simulink model "mi_modelo_MI"  (R2022b)
settings: Solver=VariableStepAuto  StartTime=0.0  StopTime=250  RelTol=1e-3
undefined symbols (not defined in the file): DiscIntNeverNeededParam, fb, fd, J, kt, Lm, Lr, Ls, Rs, sg, Tr
libraries: neural x166
(part 2 of 5)

== system mi_modelo_MI/Motor MI/landa_beta_r ==
  i_beta_s : Inport
  landa_alpha_r : Inport  Port=2
  wr : Inport  Port=3
  1/Tr : Gain  Gain=1/Tr
  Add : Sum  Inputs=++-
  Integrator : Integrator
  Lm/Tr : Gain  Gain=Lm/Tr
  Product : Product
  landa_beta_r : Outport
  wires:
  i_beta_s/1 -> Lm/Tr/1
  Integrator/1 -> landa_beta_r/1, 1/Tr/1
  wr/1 -> Product/2
  landa_alpha_r/1 -> Product/1
  Add/1 -> Integrator/1
  1/Tr/1 -> Add/3
  Lm/Tr/1 -> Add/1
  Product/1 -> Add/2

== system mi_modelo_MI/Motor MI/landa_dr ==
  i_ds : Inport
  landa_qr : Inport  Port=2
  we : Inport  Port=3
  wr : Inport  Port=4
  Gain : Gain  Gain=Lm/Tr
  Gain1 : Gain  Gain=1/Tr
  Integrator : Integrator
  Product : Product
  Subtract : Sum  Inputs=++-
  Subtract1 : Sum  Inputs=+-
  landa_dr : Outport
  wires:
  i_ds/1 -> Gain/1
  Integrator/1 -> Gain1/1, landa_dr/1
  Gain/1 -> Subtract/1
  Gain1/1 -> Subtract/3
  Subtract/1 -> Integrator/1
  landa_qr/1 -> Product/2
  Product/1 -> Subtract/2
  Subtract1/1 -> Product/1
  wr/1 -> Subtract1/2
  we/1 -> Subtract1/1

== system mi_modelo_MI/Motor MI/landa_qr ==
  i_qs : Inport
  landa_dr : Inport  Port=2
  we : Inport  Port=3
  wr : Inport  Port=4
  Gain : Gain  Gain=Lm/Tr
  Gain1 : Gain  Gain=1/Tr
  Integrator : Integrator
  Product : Product
  Subtract : Sum  Inputs=+--
  Subtract1 : Sum  Inputs=+-
  landa_qr : Outport
  wires:
  Gain1/1 -> Subtract/3
  landa_dr/1 -> Product/2
  Product/1 -> Subtract/2
  Subtract1/1 -> Product/1
  Gain/1 -> Subtract/1
  Integrator/1 -> Gain1/1, landa_qr/1
  Subtract/1 -> Integrator/1
  i_qs/1 -> Gain/1
  wr/1 -> Subtract1/2
  we/1 -> Subtract1/1

== system mi_modelo_MI/Motor MI/rotor_speed ==
  Te : Inport
  Tl : Inport  Port=2
  Gain : Gain  Gain=1/J
  Gain1 : Gain  Gain=fd
  Integrator : Integrator
  Subtract : Sum  Inputs=+--
  wr : Outport
  wires:
  Integrator/1 -> Gain1/1, wr/1
  Gain/1 -> Integrator/1
  Te/1 -> Subtract/1
  Subtract/1 -> Gain/1
  Tl/1 -> Subtract/2
  Gain1/1 -> Subtract/3

== system mi_modelo_MI/Motor MI/torque_elec ==
  landa_dr : Inport
  i_qs : Inport  Port=2
  landa_qr : Inport  Port=3
  i_ds : Inport  Port=4
  Gain : Gain  Gain=kt
  Product : Product
  Product1 : Product
  Subtract : Sum  Inputs=+-
  Te : Outport
  wires:
  i_qs/1 -> Product/2
  landa_dr/1 -> Product/1
  landa_qr/1 -> Product1/1
  i_ds/1 -> Product1/2
  Product/1 -> Subtract/1
  Product1/1 -> Subtract/2
  Gain/1 -> Te/1
  Subtract/1 -> Gain/1

== system mi_modelo_MI/NARX WR/Layer 1 ==
  "p{1}" : Inport  PortDimensions=4  SampleTime=1
      mask Display: e = 0.06;c1 = [120 230 180]/255;c2 = ([120 230 180]+0)/(256+128);c3 = ([120 230 180]+128)/(256+128);patch([0 1 1 0],[0 0 1 1],c1);patch([0 1 1 1-e 1-e 0+e],[0 0 1 1-e 0+e 0+e],c2);patch([0 0 1 1-e 0+e 0+e],[0 1 1 1-e 1-e 0+e],c3);plot([0 1 1 0 0],[0 0 1 1 0]);
  "a{2} " : Inport  Port=2  PortDimensions=1  SampleTime=1
      mask Display: e = 0.06;c1 = [120 230 180]/255;c2 = ([120 230 180]+0)/(256+128);c3 = ([120 230 180]+128)/(256+128);patch([0 1 1 0],[0 0 1 1],c1);patch([0 1 1 1-e 1-e 0+e],[0 0 1 1-e 0+e 0+e],c2);patch([0 0 1 1-e 0+e 0+e],[0 1 1 1-e 1-e 0+e],c3);plot([0 1 1 0 0],[0 0 1 1 0]);
  Delays 1 : Subsystem
      mask Display: e = 0.06;c1 = [120 150 230]/255;c2 = ([120 150 230]+0)/383;c3 = ([120 150 230]+128)/383;patch([0 1 1 0],[0 0 1 1],c1);patch([0 1 1 1-e 1-e 0+e],[0 0 1 1-e 0+e 0+e],c2);patch([0 0 1 1-e 0+e 0+e],[0 1 1 1-e 1-e 0+e],c3);plot([0 1 1 0 0],[0 0 1 1 0]);disp('1-2');
  Delays 2 : Subsystem
      mask Display: e = 0.06;c1 = [120 150 230]/255;c2 = ([120 150 230]+0)/383;c3 = ([120 150 230]+128)/383;patch([0 1 1 0],[0 0 1 1],c1);patch([0 1 1 1-e 1-e 0+e],[0 0 1 1-e 0+e 0+e],c2);patch([0 0 1 1-e 0+e 0+e],[0 1 1 1-e 1-e 0+e],c3);plot([0 1 1 0 0],[0 0 1 1 0]);disp('1-2');
  "IW{1,1}" : Subsystem
      mask Display: e = 0.06;c1 = [120 150 230]/255;c2 = ([120 150 230]+0)/383;c3 = ([120 150 230]+128)/383;patch([0 1 1 0],[0 0 1 1],c1);patch([0 1 1 1-e 1-e 0+e],[0 0 1 1-e 0+e 0+e],c2);patch([0 0 1 1-e 0+e 0+e],[0 1 1 1-e 1-e 0+e],c3);plot([0 1 1 0 0],[0 0 1 1 0]);disp('W');
  "LW{1,2}" : Subsystem
      mask Display: e = 0.06;c1 = [120 150 230]/255;c2 = ([120 150 230]+0)/383;c3 = ([120 150 230]+128)/383;patch([0 1 1 0],[0 0 1 1],c1);patch([0 1 1 1-e 1-e 0+e],[0 0 1 1-e 0+e 0+e],c2);patch([0 0 1 1-e 0+e 0+e],[0 1 1 1-e 1-e 0+e],c3);plot([0 1 1 0 0],[0 0 1 1 0]);disp('W');
  "b{1}" : Constant  Value=[-1.8998763615156166739694754141964949667453765869140625;1.7162424238927365127693747126613743603229522705078125;1.873778335719318288710155684384517371654510498046875;1.2761620955153916145974335449864156544208526611328125;-0.943914474908234435446274801506660878658294677734375;0.6149915255390541179991714670904912054538726806640625;1.2780413566537642822140696807764470577239990234375;1.01453395825711556454962192219682037830352783203125;0.842453920367021158455145268817432224750518798828125;0.73720646264958755722318528569303452968597412109375;0.4984224377356063495625448922510258853435516357421875;-0.64613247194810929929786880165920592844486236572265625;-0.1218890242028434489629518111541983671486377716064453125;0.006777158234348323873064146027900278568267822265625;-0.02844198720616673836669718866687617264688014984130859375;0.31303593350495850788917095997021533548831939697265625;-0.57699423755770595789726939983665943145751953125;0.316780417226055988066946156322956085205078125;0.68420763225480529801103557474561966955661773681640625;0.83882619819923254222970854243612848222255706787109375;0.68908943201714423221204697256325744092464447021484375;-0.79636082633369686956115174325532279908657073974609375;0.99883419950671770148886707829660736024379730224609375;-0.96148781215878909023331289063207805156707763671875;-0.888341997791541881923649270902387797832489013671875;1.134062865515947038375088595785200595855712890625;-1.5752696276526256813355075792060233652591705322265625;1.5323125142516909047429862766875885426998138427734375;1.739636071487099311383417443721555173397064208984375;-2.010421496688121312246266825241036713123321533203125]
      mask Display: e = 0.06;c1 = [120 150 230]/255;c2 = ([120 150 230]+0)/383;c3 = ([120 150 230]+128)/383;patch([0 1 1 0],[0 0 1 1],c1);patch([0 1 1 1-e 1-e 0+e],[0 0 1 1-e 0+e 0+e],c2);patch([0 0 1 1-e 0+e 0+e],[0 1 1 1-e 1-e 0+e],c3);plot([0 1 1 0 0],[0 0 1 1 0]);disp('b');
  netsum : Sum  Inputs=3  InputSameDT=on  SaturateOnIntegerOverflow=on  OutDataTypeStr=Inherit: Same as first input
      mask Display: e = 0.06;c1 = [120 150 230]/255;c2 = ([120 150 230]+0)/383;c3 = ([120 150 230]+128)/383;patch([0 1 1 0],[0 0 1 1],c1);patch([0 1 1 1-e 1-e 0+e],[0 0 1 1-e 0+e 0+e],c2);patch([0 0 1 1-e 0+e 0+e],[0 1 1 1-e 1-e 0+e],c3);plot([0 1 1 0 0],[0 0 1 1 0]);disp('+');
  tansig : neural/Transfer Functions/tansig
  "a{1}" : Outport  InitialOutput=[0;0;0;0;0;0;0;0;0;0;0;0;0;0;0;0;0;0;0;0;0;0;0;0;0;0;0;0;0;0]
      mask Display: e = 0.06;c1 = [120 230 180]/255;c2 = ([120 230 180]+0)/(256+128);c3 = ([120 230 180]+128)/(256+128);patch([0 1 1 0],[0 0 1 1],c1);patch([0 1 1 1-e 1-e 0+e],[0 0 1 1-e 0+e 0+e],c2);patch([0 0 1 1-e 0+e 0+e],[0 1 1 1-e 1-e 0+e],c3);plot([0 1 1 0 0],[0 0 1 1 0]);
  wires:
  "p{1}"/1 -> Delays 1/1("p{1}")
  Delays 1/1("pd{1,1}") -> "IW{1,1}"/1("pd{1,1}")
  "IW{1,1}"/1("iz{1,1}") -> netsum/1
  "a{2} "/1 -> Delays 2/1("p{1}")
  Delays 2/1("pd{1,2}") -> "LW{1,2}"/1("ad{1,2}")
  "LW{1,2}"/1("lz{1,2}") -> netsum/2
  "b{1}"/1 -> netsum/3
  netsum/1 -> tansig/1
  tansig/1 -> "a{1}"/1

== system mi_modelo_MI/NARX WR/Layer 2 ==
  "a{1} " : Inport  PortDimensions=30  SampleTime=1
      mask Display: e = 0.06;c1 = [120 230 180]/255;c2 = ([120 230 180]+0)/(256+128);c3 = ([120 230 180]+128)/(256+128);patch([0 1 1 0],[0 0 1 1],c1);patch([0 1 1 1-e 1-e 0+e],[0 0 1 1-e 0+e 0+e],c2);patch([0 0 1 1-e 0+e 0+e],[0 1 1 1-e 1-e 0+e],c3);plot([0 1 1 0 0],[0 0 1 1 0]);
  Delays 1 : Subsystem
      mask Display: e = 0.06;c1 = [120 150 230]/255;c2 = ([120 150 230]+0)/383;c3 = ([120 150 230]+128)/383;patch([0 1 1 0],[0 0 1 1],c1);patch([0 1 1 1-e 1-e 0+e],[0 0 1 1-e 0+e 0+e],c2);patch([0 0 1 1-e 0+e 0+e],[0 1 1 1-e 1-e 0+e],c3);plot([0 1 1 0 0],[0 0 1 1 0]);disp('0');
  "LW{2,1}" : Subsystem
      mask Display: e = 0.06;c1 = [120 150 230]/255;c2 = ([120 150 230]+0)/383;c3 = ([120 150 230]+128)/383;patch([0 1 1 0],[0 0 1 1],c1);patch([0 1 1 1-e 1-e 0+e],[0 0 1 1-e 0+e 0+e],c2);patch([0 0 1 1-e 0+e 0+e],[0 1 1 1-e 1-e 0+e],c3);plot([0 1 1 0 0],[0 0 1 1 0]);disp('W');
  "b{2}" : Constant  Value=0.2154209171011988444011109322673291899263858795166015625
      mask Display: e = 0.06;c1 = [120 150 230]/255;c2 = ([120 150 230]+0)/383;c3 = ([120 150 230]+128)/383;patch([0 1 1 0],[0 0 1 1],c1);patch([0 1 1 1-e 1-e 0+e],[0 0 1 1-e 0+e 0+e],c2);patch([0 0 1 1-e 0+e 0+e],[0 1 1 1-e 1-e 0+e],c3);plot([0 1 1 0 0],[0 0 1 1 0]);disp('b');
  netsum : Sum  Inputs=2  InputSameDT=on  SaturateOnIntegerOverflow=on  OutDataTypeStr=Inherit: Same as first input
      mask Display: e = 0.06;c1 = [120 150 230]/255;c2 = ([120 150 230]+0)/383;c3 = ([120 150 230]+128)/383;patch([0 1 1 0],[0 0 1 1],c1);patch([0 1 1 1-e 1-e 0+e],[0 0 1 1-e 0+e 0+e],c2);patch([0 0 1 1-e 0+e 0+e],[0 1 1 1-e 1-e 0+e],c3);plot([0 1 1 0 0],[0 0 1 1 0]);disp('+');
  purelin : neural/Transfer Functions/purelin
  "a{2}" : Outport  InitialOutput=0
      mask Display: e = 0.06;c1 = [120 230 180]/255;c2 = ([120 230 180]+0)/(256+128);c3 = ([120 230 180]+128)/(256+128);patch([0 1 1 0],[0 0 1 1],c1);patch([0 1 1 1-e 1-e 0+e],[0 0 1 1-e 0+e 0+e],c2);patch([0 0 1 1-e 0+e 0+e],[0 1 1 1-e 1-e 0+e],c3);plot([0 1 1 0 0],[0 0 1 1 0]);
  wires:
  "a{1} "/1 -> Delays 1/1("p{2}")
  Delays 1/1("pd{2,1}") -> "LW{2,1}"/1("ad{2,1}")
  "LW{2,1}"/1("lz{2,1}") -> netsum/1
  "b{2}"/1 -> netsum/2
  netsum/1 -> purelin/1
  purelin/1 -> "a{2}"/1

== system mi_modelo_MI/NARX WR/Process Input 1 ==
  x : Inport  PortDimensions=4  SampleTime=1
      mask Display: e = 0.06;c1 = [120 230 180]/255;c2 = ([120 230 180]+0)/(256+128);c3 = ([120 230 180]+128)/(256+128);patch([0 1 1 0],[0 0 1 1],c1);patch([0 1 1 1-e 1-e 0+e],[0 0 1 1-e 0+e 0+e],c2);patch([0 0 1 1-e 0+e 0+e],[0 1 1 1-e 1-e 0+e],c3);plot([0 1 1 0 0],[0 0 1 1 0]);
  mapminmax : neural/Processing Functions/mapminmax  xmin=[-23.2701523591743253405184077565;-23.2701524234732346485543530434;-14.6225112575844971019023432746;-14.9061771632823809596857245197]  xmax=[23.2701525537971569690398609964;23.2701525393023374022050120402;14.4575467458226949446498110774;14.8335050296775126099646513467]  ymin=-1  ymax=1
  p : Outport  PortDimensions=4  SampleTime=1
      mask Display: e = 0.06;c1 = [120 230 180]/255;c2 = ([120 230 180]+0)/(256+128);c3 = ([120 230 180]+128)/(256+128);patch([0 1 1 0],[0 0 1 1],c1);patch([0 1 1 1-e 1-e 0+e],[0 0 1 1-e 0+e 0+e],c2);patch([0 0 1 1-e 0+e 0+e],[0 1 1 1-e 1-e 0+e],c3);plot([0 1 1 0 0],[0 0 1 1 0]);
  wires:
  x/1 -> mapminmax/1
  mapminmax/1 -> p/1

== system mi_modelo_MI/NARX WR/Process Output 1 ==
  a : Inport  PortDimensions=1  SampleTime=1
      mask Display: e = 0.06;c1 = [120 230 180]/255;c2 = ([120 230 180]+0)/(256+128);c3 = ([120 230 180]+128)/(256+128);patch([0 1 1 0],[0 0 1 1],c1);patch([0 1 1 1-e 1-e 0+e],[0 0 1 1-e 0+e 0+e],c2);patch([0 0 1 1-e 0+e 0+e],[0 1 1 1-e 1-e 0+e],c3);plot([0 1 1 0 0],[0 0 1 1 0]);
  mapminmax_reverse : neural/Processing Functions/mapminmax_reverse  xmin=-9.70936783596300934107148350449  xmax=9.91950848181129529734789684881  ymin=-1  ymax=1
  y : Outport  PortDimensions=1  SampleTime=1
      mask Display: e = 0.06;c1 = [120 230 180]/255;c2 = ([120 230 180]+0)/(256+128);c3 = ([120 230 180]+128)/(256+128);patch([0 1 1 0],[0 0 1 1],c1);patch([0 1 1 1-e 1-e 0+e],[0 0 1 1-e 0+e 0+e],c2);patch([0 0 1 1-e 0+e 0+e],[0 1 1 1-e 1-e 0+e],c3);plot([0 1 1 0 0],[0 0 1 1 0]);
  wires:
  a/1 -> mapminmax_reverse/1
  mapminmax_reverse/1 -> y/1

== system mi_modelo_MI/FFNN FluxRotor/Layer 1/Delays 1 ==
  "p{1}" : Inport  PortDimensions=5
      mask Display: e = 0.06;c1 = [120 230 180]/255;c2 = ([120 230 180]+0)/(256+128);c3 = ([120 230 180]+128)/(256+128);patch([0 1 1 0],[0 0 1 1],c1);patch([0 1 1 1-e 1-e 0+e],[0 0 1 1-e 0+e 0+e],c2);patch([0 0 1 1-e 0+e 0+e],[0 1 1 1-e 1-e 0+e],c3);plot([0 1 1 0 0],[0 0 1 1 0]);
  mux : Mux  Inputs=1
      mask Display: e = 0.06;c1 = [120 150 230]/255;c2 = ([120 150 230]+0)/383;c3 = ([120 150 230]+128)/383;patch([0 1 1 0],[0 0 1 1],c1);patch([0 1 1 1-e 1-e 0+e],[0 0 1 1-e 0+e 0+e],c2);patch([0 0 1 1-e 0+e 0+e],[0 1 1 1-e 1-e 0+e],c3);plot([0 1 1 0 0],[0 0 1 1 0]);disp('Mux')
  "pd{1,1}" : Outport
      mask Display: e = 0.06;c1 = [120 230 180]/255;c2 = ([120 230 180]+0)/(256+128);c3 = ([120 230 180]+128)/(256+128);patch([0 1 1 0],[0 0 1 1],c1);patch([0 1 1 1-e 1-e 0+e],[0 0 1 1-e 0+e 0+e],c2);patch([0 0 1 1-e 0+e 0+e],[0 1 1 1-e 1-e 0+e],c3);plot([0 1 1 0 0],[0 0 1 1 0]);
  wires:
  "p{1}"/1 -> mux/1
  mux/1 -> "pd{1,1}"/1

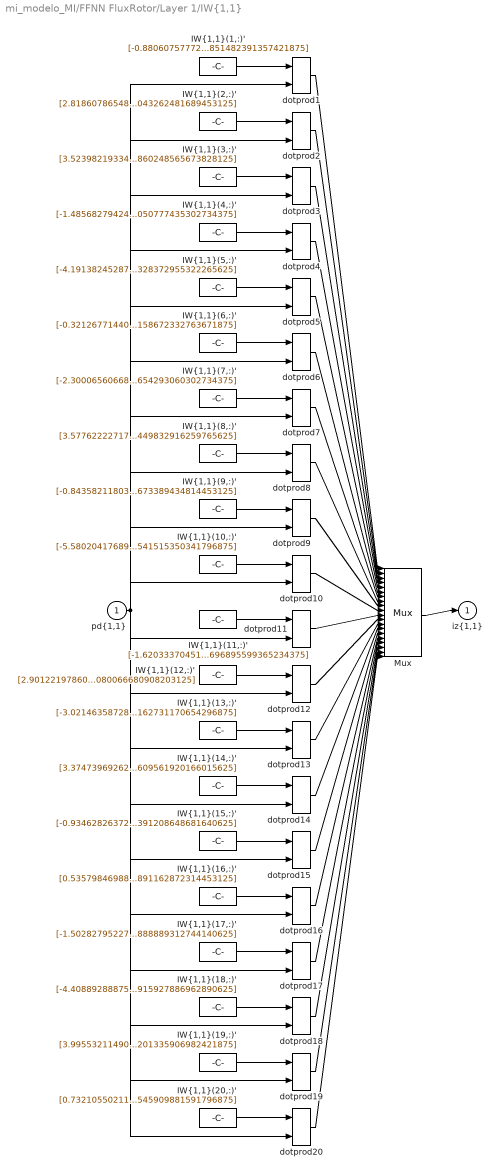
== system mi_modelo_MI/FFNN FluxRotor/Layer 1/IW{1,1} ==
  "pd{1,1}" : Inport  PortDimensions=5
      mask Display: e = 0.06;c1 = [120 230 180]/255;c2 = ([120 230 180]+0)/(256+128);c3 = ([120 230 180]+128)/(256+128);patch([0 1 1 0],[0 0 1 1],c1);patch([0 1 1 1-e 1-e 0+e],[0 0 1 1-e 0+e 0+e],c2);patch([0 0 1 1-e 0+e 0+e],[0 1 1 1-e 1-e 0+e],c3);plot([0 1 1 0 0],[0 0 1 1 0]);
  "IW{1,1}(1,:)'" : Constant  Value=[-0.880607577720789347353047560318373143672943115234375;-4.66559308676044270924876400385983288288116455078125;-1.0483518811015446470236156528699211776256561279296875;6.68023141628481198495137505233287811279296875;-0.0240170286331755356012962465683813206851482391357421875]
      mask Display: e = 0.06;c1 = [120 150 230]/255;c2 = ([120 150 230]+0)/383;c3 = ([120 150 230]+128)/383;patch([0 1 1 0],[0 0 1 1],c1);patch([0 1 1 1-e 1-e 0+e],[0 0 1 1-e 0+e 0+e],c2);patch([0 0 1 1-e 0+e 0+e],[0 1 1 1-e 1-e 0+e],c3);plot([0 1 1 0 0],[0 0 1 1 0]);disp('Weights');
  "IW{1,1}(10,:)'" : Constant  Value=[-5.58020417689812830985829350538551807403564453125;-2.275638438988880185576135772862471640110015869140625;6.47800315456226005750295371399261057376861572265625;2.344852971662279461639855071553029119968414306640625;0.65234850837414615210008150825160555541515350341796875]
      mask Display: e = 0.06;c1 = [120 150 230]/255;c2 = ([120 150 230]+0)/383;c3 = ([120 150 230]+128)/383;patch([0 1 1 0],[0 0 1 1],c1);patch([0 1 1 1-e 1-e 0+e],[0 0 1 1-e 0+e 0+e],c2);patch([0 0 1 1-e 0+e 0+e],[0 1 1 1-e 1-e 0+e],c3);plot([0 1 1 0 0],[0 0 1 1 0]);disp('Weights');
  "IW{1,1}(11,:)'" : Constant  Value=[-1.6203337045151666728770578629337251186370849609375;2.56791490274778855251724962727166712284088134765625;2.95917854989119177844258956611156463623046875;-3.1891740599872395733882513013668358325958251953125;-1.256089823357095180966780390008352696895599365234375]
      mask Display: e = 0.06;c1 = [120 150 230]/255;c2 = ([120 150 230]+0)/383;c3 = ([120 150 230]+128)/383;patch([0 1 1 0],[0 0 1 1],c1);patch([0 1 1 1-e 1-e 0+e],[0 0 1 1-e 0+e 0+e],c2);patch([0 0 1 1-e 0+e 0+e],[0 1 1 1-e 1-e 0+e],c3);plot([0 1 1 0 0],[0 0 1 1 0]);disp('Weights');
  "IW{1,1}(12,:)'" : Constant  Value=[2.901221978601477236026084938202984631061553955078125;6.35169355116053058196712299832142889499664306640625;-3.613441479298154401789133771671913564205169677734375;-7.422646017895232262162608094513416290283203125;5.50138379513384467855985349160619080066680908203125]
      mask Display: e = 0.06;c1 = [120 150 230]/255;c2 = ([120 150 230]+0)/383;c3 = ([120 150 230]+128)/383;patch([0 1 1 0],[0 0 1 1],c1);patch([0 1 1 1-e 1-e 0+e],[0 0 1 1-e 0+e 0+e],c2);patch([0 0 1 1-e 0+e 0+e],[0 1 1 1-e 1-e 0+e],c3);plot([0 1 1 0 0],[0 0 1 1 0]);disp('Weights');
  "IW{1,1}(13,:)'" : Constant  Value=[-3.02146358728570607610208753612823784351348876953125;-4.8228675598348100805878857499919831752777099609375;3.81877645756408679034166198107413947582244873046875;5.87144628057232953466382241458632051944732666015625;-4.8366977902518026866118816542439162731170654296875]
      mask Display: e = 0.06;c1 = [120 150 230]/255;c2 = ([120 150 230]+0)/383;c3 = ([120 150 230]+128)/383;patch([0 1 1 0],[0 0 1 1],c1);patch([0 1 1 1-e 1-e 0+e],[0 0 1 1-e 0+e 0+e],c2);patch([0 0 1 1-e 0+e 0+e],[0 1 1 1-e 1-e 0+e],c3);plot([0 1 1 0 0],[0 0 1 1 0]);disp('Weights');
  "IW{1,1}(14,:)'" : Constant  Value=[3.374739692625540410375606370507739484310150146484375;3.339377074449438875802798065706156194210052490234375;-3.5654861463754077277599208173342049121856689453125;-3.026737387277985913414113383623771369457244873046875;-1.925186125287125182836689418763853609561920166015625]
      mask Display: e = 0.06;c1 = [120 150 230]/255;c2 = ([120 150 230]+0)/383;c3 = ([120 150 230]+128)/383;patch([0 1 1 0],[0 0 1 1],c1);patch([0 1 1 1-e 1-e 0+e],[0 0 1 1-e 0+e 0+e],c2);patch([0 0 1 1-e 0+e 0+e],[0 1 1 1-e 1-e 0+e],c3);plot([0 1 1 0 0],[0 0 1 1 0]);disp('Weights');
  "IW{1,1}(15,:)'" : Constant  Value=[-0.93462826372438934097175433635129593312740325927734375;-3.998741084281752566909062807098962366580963134765625;1.2145989900400682159897769452072679996490478515625;4.1364519411066975607127460534684360027313232421875;-2.493457984136628002858060426660813391208648681640625]
      mask Display: e = 0.06;c1 = [120 150 230]/255;c2 = ([120 150 230]+0)/383;c3 = ([120 150 230]+128)/383;patch([0 1 1 0],[0 0 1 1],c1);patch([0 1 1 1-e 1-e 0+e],[0 0 1 1-e 0+e 0+e],c2);patch([0 0 1 1-e 0+e 0+e],[0 1 1 1-e 1-e 0+e],c3);plot([0 1 1 0 0],[0 0 1 1 0]);disp('Weights');
  "IW{1,1}(16,:)'" : Constant  Value=[0.5357984698861371075651049977750517427921295166015625;-2.62158945848266267120152406278066337108612060546875;0.0606042943991576821272104780291556380689144134521484375;2.9951828590030391552545552258379757404327392578125;1.936298560391311429640381902572698891162872314453125]
      mask Display: e = 0.06;c1 = [120 150 230]/255;c2 = ([120 150 230]+0)/383;c3 = ([120 150 230]+128)/383;patch([0 1 1 0],[0 0 1 1],c1);patch([0 1 1 1-e 1-e 0+e],[0 0 1 1-e 0+e 0+e],c2);patch([0 0 1 1-e 0+e 0+e],[0 1 1 1-e 1-e 0+e],c3);plot([0 1 1 0 0],[0 0 1 1 0]);disp('Weights');
  "IW{1,1}(17,:)'" : Constant  Value=[-1.50282795227539356375245915842242538928985595703125;-0.11842576597614247468914783212312613613903522491455078125;2.366553450648900547292896590079180896282196044921875;-0.215949957821690963211125335874385200440883636474609375;-0.78467129817601988239772481392719782888889312744140625]
      mask Display: e = 0.06;c1 = [120 150 230]/255;c2 = ([120 150 230]+0)/383;c3 = ([120 150 230]+128)/383;patch([0 1 1 0],[0 0 1 1],c1);patch([0 1 1 1-e 1-e 0+e],[0 0 1 1-e 0+e 0+e],c2);patch([0 0 1 1-e 0+e 0+e],[0 1 1 1-e 1-e 0+e],c3);plot([0 1 1 0 0],[0 0 1 1 0]);disp('Weights');
  "IW{1,1}(18,:)'" : Constant  Value=[-4.4088928887596399164294780348427593708038330078125;-3.400205713156308373612546347430907189846038818359375;4.9218386962876099488539693993516266345977783203125;4.79125627925675789953174898982979357242584228515625;1.57228301933683045632506036781705915927886962890625]
      mask Display: e = 0.06;c1 = [120 150 230]/255;c2 = ([120 150 230]+0)/383;c3 = ([120 150 230]+128)/383;patch([0 1 1 0],[0 0 1 1],c1);patch([0 1 1 1-e 1-e 0+e],[0 0 1 1-e 0+e 0+e],c2);patch([0 0 1 1-e 0+e 0+e],[0 1 1 1-e 1-e 0+e],c3);plot([0 1 1 0 0],[0 0 1 1 0]);disp('Weights');
  "IW{1,1}(19,:)'" : Constant  Value=[3.995532114901846565402365740737877786159515380859375;2.166128519502908300609078651177696883678436279296875;-4.489432754628733590607225778512656688690185546875;-2.059827883364778511321446785586886107921600341796875;-0.65104897333927957969734734433586709201335906982421875]
      mask Display: e = 0.06;c1 = [120 150 230]/255;c2 = ([120 150 230]+0)/383;c3 = ([120 150 230]+128)/383;patch([0 1 1 0],[0 0 1 1],c1);patch([0 1 1 1-e 1-e 0+e],[0 0 1 1-e 0+e 0+e],c2);patch([0 0 1 1-e 0+e 0+e],[0 1 1 1-e 1-e 0+e],c3);plot([0 1 1 0 0],[0 0 1 1 0]);disp('Weights');
  "IW{1,1}(2,:)'" : Constant  Value=[2.81860786548738762036236948915757238864898681640625;-1.4151144856359672008494499095831997692584991455078125;-1.9708719877646638796164779705577529966831207275390625;1.534668662772387559556364067248068749904632568359375;-2.729902015750913069069838456925936043262481689453125]
      mask Display: e = 0.06;c1 = [120 150 230]/255;c2 = ([120 150 230]+0)/383;c3 = ([120 150 230]+128)/383;patch([0 1 1 0],[0 0 1 1],c1);patch([0 1 1 1-e 1-e 0+e],[0 0 1 1-e 0+e 0+e],c2);patch([0 0 1 1-e 0+e 0+e],[0 1 1 1-e 1-e 0+e],c3);plot([0 1 1 0 0],[0 0 1 1 0]);disp('Weights');
  "IW{1,1}(20,:)'" : Constant  Value=[0.7321055021183997535416665414231829345226287841796875;0.87735966003277543467930854603764601051807403564453125;0.039463194394777689755215988043346442282199859619140625;-1.98217512800962847308028358384035527706146240234375;1.2592924569731269723860123121994547545909881591796875]
      mask Display: e = 0.06;c1 = [120 150 230]/255;c2 = ([120 150 230]+0)/383;c3 = ([120 150 230]+128)/383;patch([0 1 1 0],[0 0 1 1],c1);patch([0 1 1 1-e 1-e 0+e],[0 0 1 1-e 0+e 0+e],c2);patch([0 0 1 1-e 0+e 0+e],[0 1 1 1-e 1-e 0+e],c3);plot([0 1 1 0 0],[0 0 1 1 0]);disp('Weights');
  "IW{1,1}(3,:)'" : Constant  Value=[3.5239821933432846634559609810821712017059326171875;1.491994731512176652898915563127957284450531005859375;-4.5384749005171673985614688717760145664215087890625;-3.65705337101311034331274640862829983234405517578125;0.2174859456841918003977554008088191039860248565673828125]
      mask Display: e = 0.06;c1 = [120 150 230]/255;c2 = ([120 150 230]+0)/383;c3 = ([120 150 230]+128)/383;patch([0 1 1 0],[0 0 1 1],c1);patch([0 1 1 1-e 1-e 0+e],[0 0 1 1-e 0+e 0+e],c2);patch([0 0 1 1-e 0+e 0+e],[0 1 1 1-e 1-e 0+e],c3);plot([0 1 1 0 0],[0 0 1 1 0]);disp('Weights');
  "IW{1,1}(4,:)'" : Constant  Value=[-1.4856827942488928240294399074628017842769622802734375;3.126691771181957069103418689337559044361114501953125;1.0801766325686703584807446532067842781543731689453125;-3.82571751464590281699429397122003138065338134765625;-2.171404828124730013172438702895306050777435302734375]
      mask Display: e = 0.06;c1 = [120 150 230]/255;c2 = ([120 150 230]+0)/383;c3 = ([120 150 230]+128)/383;patch([0 1 1 0],[0 0 1 1],c1);patch([0 1 1 1-e 1-e 0+e],[0 0 1 1-e 0+e 0+e],c2);patch([0 0 1 1-e 0+e 0+e],[0 1 1 1-e 1-e 0+e],c3);plot([0 1 1 0 0],[0 0 1 1 0]);disp('Weights');
  "IW{1,1}(5,:)'" : Constant  Value=[-4.19138245287409194617112007108516991138458251953125;-5.441057312013729330146816209889948368072509765625;4.92609220581658657778234555735252797603607177734375;7.0309120539422682583108326070941984653472900390625;-1.515596648404287094535902724601328372955322265625]
      mask Display: e = 0.06;c1 = [120 150 230]/255;c2 = ([120 150 230]+0)/383;c3 = ([120 150 230]+128)/383;patch([0 1 1 0],[0 0 1 1],c1);patch([0 1 1 1-e 1-e 0+e],[0 0 1 1-e 0+e 0+e],c2);patch([0 0 1 1-e 0+e 0+e],[0 1 1 1-e 1-e 0+e],c3);plot([0 1 1 0 0],[0 0 1 1 0]);disp('Weights');
  "IW{1,1}(6,:)'" : Constant  Value=[-0.321267714405825077772504982931423000991344451904296875;-3.0579108353476502912826617830432951450347900390625;-0.1650089527271223488469331641681492328643798828125;3.99918354794704544730166162480600178241729736328125;1.6555904284616189681145215217838995158672332763671875]
      mask Display: e = 0.06;c1 = [120 150 230]/255;c2 = ([120 150 230]+0)/383;c3 = ([120 150 230]+128)/383;patch([0 1 1 0],[0 0 1 1],c1);patch([0 1 1 1-e 1-e 0+e],[0 0 1 1-e 0+e 0+e],c2);patch([0 0 1 1-e 0+e 0+e],[0 1 1 1-e 1-e 0+e],c3);plot([0 1 1 0 0],[0 0 1 1 0]);disp('Weights');
  "IW{1,1}(7,:)'" : Constant  Value=[-2.300065606685610219983573188073933124542236328125;0.8157406234514847920280544713023118674755096435546875;2.284603115065495071434042984037660062313079833984375;-1.202223950632307580832502935663796961307525634765625;-1.876322561213180417638568542315624654293060302734375]
      mask Display: e = 0.06;c1 = [120 150 230]/255;c2 = ([120 150 230]+0)/383;c3 = ([120 150 230]+128)/383;patch([0 1 1 0],[0 0 1 1],c1);patch([0 1 1 1-e 1-e 0+e],[0 0 1 1-e 0+e 0+e],c2);patch([0 0 1 1-e 0+e 0+e],[0 1 1 1-e 1-e 0+e],c3);plot([0 1 1 0 0],[0 0 1 1 0]);disp('Weights');
  "IW{1,1}(8,:)'" : Constant  Value=[3.577622227178220981613776530139148235321044921875;-2.42588459093870678628945825039409101009368896484375;-3.156837934109276044836178698460571467876434326171875;2.97512286657441915593835801701061427593231201171875;-2.843299941820012666227057707146741449832916259765625]
      mask Display: e = 0.06;c1 = [120 150 230]/255;c2 = ([120 150 230]+0)/383;c3 = ([120 150 230]+128)/383;patch([0 1 1 0],[0 0 1 1],c1);patch([0 1 1 1-e 1-e 0+e],[0 0 1 1-e 0+e 0+e],c2);patch([0 0 1 1-e 0+e 0+e],[0 1 1 1-e 1-e 0+e],c3);plot([0 1 1 0 0],[0 0 1 1 0]);disp('Weights');
  "IW{1,1}(9,:)'" : Constant  Value=[-0.8435821180372109484579823401872999966144561767578125;-0.60798340647440907158483014427474699914455413818359375;0.65261208262402081725639391152071766555309295654296875;1.807597073962215805664754952886141836643218994140625;-0.23496835258478132590909126520273275673389434814453125]
      mask Display: e = 0.06;c1 = [120 150 230]/255;c2 = ([120 150 230]+0)/383;c3 = ([120 150 230]+128)/383;patch([0 1 1 0],[0 0 1 1],c1);patch([0 1 1 1-e 1-e 0+e],[0 0 1 1-e 0+e 0+e],c2);patch([0 0 1 1-e 0+e 0+e],[0 1 1 1-e 1-e 0+e],c3);plot([0 1 1 0 0],[0 0 1 1 0]);disp('Weights');
  Mux : Mux  Inputs=20
      mask Display: e = 0.06;c1 = [120 150 230]/255;c2 = ([120 150 230]+0)/383;c3 = ([120 150 230]+128)/383;patch([0 1 1 0],[0 0 1 1],c1);patch([0 1 1 1-e 1-e 0+e],[0 0 1 1-e 0+e 0+e],c2);patch([0 0 1 1-e 0+e 0+e],[0 1 1 1-e 1-e 0+e],c3);plot([0 1 1 0 0],[0 0 1 1 0]);disp('Mux');
  dotprod{1..20} (20 alike) : neural/Weight Functions/dotprod
  "iz{1,1}" : Outport
      mask Display: e = 0.06;c1 = [120 230 180]/255;c2 = ([120 230 180]+0)/(256+128);c3 = ([120 230 180]+128)/(256+128);patch([0 1 1 0],[0 0 1 1],c1);patch([0 1 1 1-e 1-e 0+e],[0 0 1 1-e 0+e 0+e],c2);patch([0 0 1 1-e 0+e 0+e],[0 1 1 1-e 1-e 0+e],c3);plot([0 1 1 0 0],[0 0 1 1 0]);
  wires:
  "IW{1,1}(1,:)'"/1 -> dotprod1/1
  "pd{1,1}"/1 -> dotprod1/2, dotprod2/2, dotprod3/2, dotprod4/2, dotprod5/2, dotprod6/2, dotprod7/2, dotprod8/2, dotprod9/2, dotprod10/2, dotprod11/2, dotprod12/2, dotprod13/2, dotprod14/2, dotprod15/2, dotprod16/2, dotprod17/2, dotprod18/2, dotprod19/2, dotprod20/2
  dotprod1/1 -> Mux/1
  "IW{1,1}(2,:)'"/1 -> dotprod2/1
  dotprod2/1 -> Mux/2
  "IW{1,1}(3,:)'"/1 -> dotprod3/1
  dotprod3/1 -> Mux/3
  "IW{1,1}(4,:)'"/1 -> dotprod4/1
  dotprod4/1 -> Mux/4
  "IW{1,1}(5,:)'"/1 -> dotprod5/1
  dotprod5/1 -> Mux/5
  "IW{1,1}(6,:)'"/1 -> dotprod6/1
  dotprod6/1 -> Mux/6
  "IW{1,1}(7,:)'"/1 -> dotprod7/1
  dotprod7/1 -> Mux/7
  "IW{1,1}(8,:)'"/1 -> dotprod8/1
  dotprod8/1 -> Mux/8
  "IW{1,1}(9,:)'"/1 -> dotprod9/1
  dotprod9/1 -> Mux/9
  "IW{1,1}(10,:)'"/1 -> dotprod10/1
  dotprod10/1 -> Mux/10
  "IW{1,1}(11,:)'"/1 -> dotprod11/1
  dotprod11/1 -> Mux/11
  "IW{1,1}(12,:)'"/1 -> dotprod12/1
  dotprod12/1 -> Mux/12
  "IW{1,1}(13,:)'"/1 -> dotprod13/1
  dotprod13/1 -> Mux/13
  "IW{1,1}(14,:)'"/1 -> dotprod14/1
  dotprod14/1 -> Mux/14
  "IW{1,1}(15,:)'"/1 -> dotprod15/1
  dotprod15/1 -> Mux/15
  "IW{1,1}(16,:)'"/1 -> dotprod16/1
  dotprod16/1 -> Mux/16
  "IW{1,1}(17,:)'"/1 -> dotprod17/1
  dotprod17/1 -> Mux/17
  "IW{1,1}(18,:)'"/1 -> dotprod18/1
  dotprod18/1 -> Mux/18
  "IW{1,1}(19,:)'"/1 -> dotprod19/1
  dotprod19/1 -> Mux/19
  "IW{1,1}(20,:)'"/1 -> dotprod20/1
  dotprod20/1 -> Mux/20
  Mux/1 -> "iz{1,1}"/1

== system mi_modelo_MI/FFNN FluxRotor/Layer 2/Delays 1 ==
  "p{2}" : Inport  PortDimensions=20
      mask Display: e = 0.06;c1 = [120 230 180]/255;c2 = ([120 230 180]+0)/(256+128);c3 = ([120 230 180]+128)/(256+128);patch([0 1 1 0],[0 0 1 1],c1);patch([0 1 1 1-e 1-e 0+e],[0 0 1 1-e 0+e 0+e],c2);patch([0 0 1 1-e 0+e 0+e],[0 1 1 1-e 1-e 0+e],c3);plot([0 1 1 0 0],[0 0 1 1 0]);
  mux : Mux  Inputs=1
      mask Display: e = 0.06;c1 = [120 150 230]/255;c2 = ([120 150 230]+0)/383;c3 = ([120 150 230]+128)/383;patch([0 1 1 0],[0 0 1 1],c1);patch([0 1 1 1-e 1-e 0+e],[0 0 1 1-e 0+e 0+e],c2);patch([0 0 1 1-e 0+e 0+e],[0 1 1 1-e 1-e 0+e],c3);plot([0 1 1 0 0],[0 0 1 1 0]);disp('Mux')
  "pd{2,1}" : Outport
      mask Display: e = 0.06;c1 = [120 230 180]/255;c2 = ([120 230 180]+0)/(256+128);c3 = ([120 230 180]+128)/(256+128);patch([0 1 1 0],[0 0 1 1],c1);patch([0 1 1 1-e 1-e 0+e],[0 0 1 1-e 0+e 0+e],c2);patch([0 0 1 1-e 0+e 0+e],[0 1 1 1-e 1-e 0+e],c3);plot([0 1 1 0 0],[0 0 1 1 0]);
  wires:
  "p{2}"/1 -> mux/1
  mux/1 -> "pd{2,1}"/1

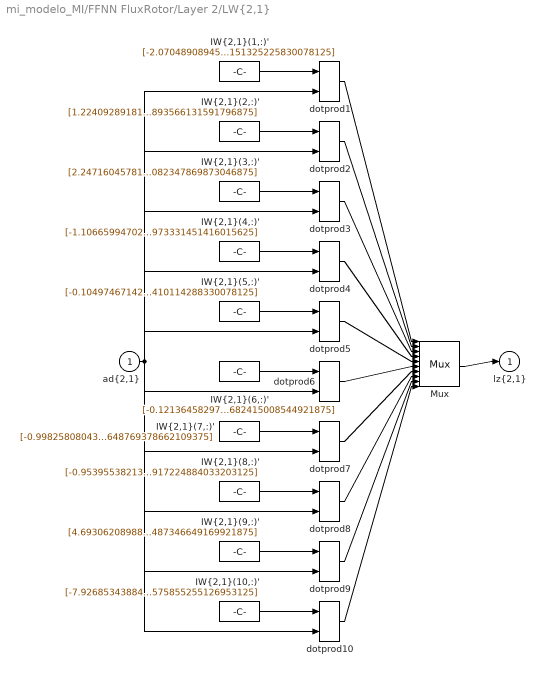
== system mi_modelo_MI/FFNN FluxRotor/Layer 2/LW{2,1} ==
  "ad{2,1}" : Inport  PortDimensions=20
      mask Display: e = 0.06;c1 = [120 230 180]/255;c2 = ([120 230 180]+0)/(256+128);c3 = ([120 230 180]+128)/(256+128);patch([0 1 1 0],[0 0 1 1],c1);patch([0 1 1 1-e 1-e 0+e],[0 0 1 1-e 0+e 0+e],c2);patch([0 0 1 1-e 0+e 0+e],[0 1 1 1-e 1-e 0+e],c3);plot([0 1 1 0 0],[0 0 1 1 0]);
  "IW{2,1}(1,:)'" : Constant  Value=[-2.0704890894578422688709906651638448238372802734375;0.1667525302340492621144818485845462419092655181884765625;1.97394608542951477403448734548874199390411376953125;-0.70177730140386784807304820787976495921611785888671875;-0.5145579737792378427485573411104269325733184814453125;-3.123678174178020849893755439552478492259979248046875;-1.7519571403207956361569586078985594213008880615234375;0.206875768927555270249030172635684721171855926513671875;6.2633595522501028796114042052067816257476806640625;-1.0335110823648527844653699503396637737751007080078125;-4.32570071698872649079703478491865098476409912109375;-0.8247531956975733269388229018659330904483795166015625;-0.304228730691319615431211786926724016666412353515625;-2.280971073495023038191220621229149401187896728515625;-1.28725637392227110211706531117670238018035888671875;-0.228162413595962565437957891845144331455230712890625;6.2588570094573210411681429832242429256439208984375;-1.3280433107389324476343972492031753063201904296875;-2.6294110420783933790289665921591222286224365234375;-0.39836946489601665621904658109997399151325225830078125]
      mask Display: e = 0.06;c1 = [120 150 230]/255;c2 = ([120 150 230]+0)/383;c3 = ([120 150 230]+128)/383;patch([0 1 1 0],[0 0 1 1],c1);patch([0 1 1 1-e 1-e 0+e],[0 0 1 1-e 0+e 0+e],c2);patch([0 0 1 1-e 0+e 0+e],[0 1 1 1-e 1-e 0+e],c3);plot([0 1 1 0 0],[0 0 1 1 0]);disp('weights');
  "IW{2,1}(10,:)'" : Constant  Value=[-7.92685343884219406618285574950277805328369140625;11.5953080425571357636727043427526950836181640625;6.12476854477429100143126561306416988372802734375;3.75231396991518639794094269745983183383941650390625;8.4678835110283383613705154857598245143890380859375;10.6193824426408287564527199720032513141632080078125;16.2701788565038469869250548072159290313720703125;-9.632985372968395409998265677131712436676025390625;4.24610293013653272709007069352082908153533935546875;-4.63713063886268361812881266814656555652618408203125;9.6223125310952610789172467775642871856689453125;6.947020841916327071885461919009685516357421875;8.37924958138606967850137152709066867828369140625;-7.4452602444672013604076710180379450321197509765625;-4.17591395056241498906501874444074928760528564453125;10.93652905331992997162160463631153106689453125;-10.805677227781220750557622523047029972076416015625;-7.26363334833022822323300715652294456958770751953125;8.665587848570577733653408358804881572723388671875;1.74977938378019093335069555905647575855255126953125]
      mask Display: e = 0.06;c1 = [120 150 230]/255;c2 = ([120 150 230]+0)/383;c3 = ([120 150 230]+128)/383;patch([0 1 1 0],[0 0 1 1],c1);patch([0 1 1 1-e 1-e 0+e],[0 0 1 1-e 0+e 0+e],c2);patch([0 0 1 1-e 0+e 0+e],[0 1 1 1-e 1-e 0+e],c3);plot([0 1 1 0 0],[0 0 1 1 0]);disp('weights');
  "IW{2,1}(2,:)'" : Constant  Value=[1.2240928918117470747262132135801948606967926025390625;0.01472155349115846119378847589587167021818459033966064453125;-1.36183985673352214718079267186112701892852783203125;-0.5483825553851773282332260350813157856464385986328125;-0.66965298543409679243865184616879560053348541259765625;3.041628692462564398368840556940995156764984130859375;1.5911111210427988371662877398193813860416412353515625;0.58237695293281499520077204579138197004795074462890625;-3.14769721342846420242267413414083421230316162109375;-0.6119224268464245053422700948431156575679779052734375;2.82445835550846791051071704714559018611907958984375;0.2399316562220478454836580795017653144896030426025390625;-0.317258617248349750195046681255917064845561981201171875;1.5364558486762016631388405585312284529209136962890625;-0.99537051755187844204186831120750866830348968505859375;-0.348553149801896611226226241342374123632907867431640625;-1.2731307862400778052602845491492189466953277587890625;-0.976898213333363241162032863940112292766571044921875;-1.3063780768985377989110929775051772594451904296875;-0.75240354646783191849834793174522928893566131591796875]
      mask Display: e = 0.06;c1 = [120 150 230]/255;c2 = ([120 150 230]+0)/383;c3 = ([120 150 230]+128)/383;patch([0 1 1 0],[0 0 1 1],c1);patch([0 1 1 1-e 1-e 0+e],[0 0 1 1-e 0+e 0+e],c2);patch([0 0 1 1-e 0+e 0+e],[0 1 1 1-e 1-e 0+e],c3);plot([0 1 1 0 0],[0 0 1 1 0]);disp('weights');
  "IW{2,1}(3,:)'" : Constant  Value=[2.247160457814395773112892129574902355670928955078125;-1.5794138989353101454327088504214771091938018798828125;-2.272877231487738125537134692422114312648773193359375;0.1149061714597417738215057170236832462251186370849609375;0.413338037912433897691499851134722121059894561767578125;2.29888914102615782297789337462745606899261474609375;1.655626530703173227010438495199196040630340576171875;1.8206622757850039473481729146442376077175140380859375;-5.0831954838007593622251079068519175052642822265625;1.6447324393223039518119321655831299722194671630859375;1.39102760111468537473911055712960660457611083984375;-2.45372094073252444701438435004092752933502197265625;-3.241991066219716888241464403108693659305572509765625;1.76219217490739143983091707923449575901031494140625;1.08818618411190559669421418220736086368560791015625;0.01397779281263417973379947767398334690369665622711181640625;-2.058785043624947519447232480160892009735107421875;0.78734447619881897661997527393396012485027313232421875;3.657661588212008485498927257140167057514190673828125;-0.00634156051072968900139681380778711172752082347869873046875]
      mask Display: e = 0.06;c1 = [120 150 230]/255;c2 = ([120 150 230]+0)/383;c3 = ([120 150 230]+128)/383;patch([0 1 1 0],[0 0 1 1],c1);patch([0 1 1 1-e 1-e 0+e],[0 0 1 1-e 0+e 0+e],c2);patch([0 0 1 1-e 0+e 0+e],[0 1 1 1-e 1-e 0+e],c3);plot([0 1 1 0 0],[0 0 1 1 0]);disp('weights');
  "IW{2,1}(4,:)'" : Constant  Value=[-1.1066599470271991645375919688376598060131072998046875;0.5196017227931448712041628823499195277690887451171875;0.2021582012449442411483602199950837530195713043212890625;-0.1295138878071091792509861306825769133865833282470703125;-0.49675655908795557369472817299538291990756988525390625;-2.08435358993625019508044715621508657932281494140625;-4.57075762025845921954214645666070282459259033203125;-2.179910026099734832172316600917838513851165771484375;-0.0180135367304478342942442026242133579216897487640380859375;2.011115709295444364812510684714652597904205322265625;-1.399401638562465688409020003746263682842254638671875;1.8397622301123359722652139680576510727405548095703125;2.007070867606020048157233759411610662937164306640625;0.8259068174838131159987142382306046783924102783203125;1.307721025575197426604745487566106021404266357421875;-3.542307156139337553923951418255455791950225830078125;1.5053401231993912556816894721123389899730682373046875;2.64886520125326097030438177171163260936737060546875;1.1474291752277701039730573029373772442340850830078125;4.60210540847337856718013426871038973331451416015625]
      mask Display: e = 0.06;c1 = [120 150 230]/255;c2 = ([120 150 230]+0)/383;c3 = ([120 150 230]+128)/383;patch([0 1 1 0],[0 0 1 1],c1);patch([0 1 1 1-e 1-e 0+e],[0 0 1 1-e 0+e 0+e],c2);patch([0 0 1 1-e 0+e 0+e],[0 1 1 1-e 1-e 0+e],c3);plot([0 1 1 0 0],[0 0 1 1 0]);disp('weights');
  "IW{2,1}(5,:)'" : Constant  Value=[-0.10497467142051920829803890455877990461885929107666015625;-2.16034347238769175447714587789960205554962158203125;0.2420535347874800125023142527425079606473445892333984375;-3.310554960323522255549733017687685787677764892578125;-1.500621643960166284870183517341502010822296142578125;-0.58251109481545293444781918879016302525997161865234375;-0.598401669611262843062604588340036571025848388671875;2.328475054213329453745018327026627957820892333984375;0.4520662806906994291011869790963828563690185546875;3.026687126740649436129615423851646482944488525390625;-2.591704460962274136903715771040879189968109130859375;-3.751648161520083846198758692480623722076416015625;-4.493074863069569602203046088106930255889892578125;-0.142900400999991961104029769558110274374485015869140625;2.75439242616482005132638732902705669403076171875;-3.420159550133089254586593597196042537689208984375;0.62841959016446657937393638349021784961223602294921875;-0.4419154497349009336204517239821143448352813720703125;3.28963559963195617541487081325612962245941162109375;1.2287806410384256583512296856497414410114288330078125]
      mask Display: e = 0.06;c1 = [120 150 230]/255;c2 = ([120 150 230]+0)/383;c3 = ([120 150 230]+128)/383;patch([0 1 1 0],[0 0 1 1],c1);patch([0 1 1 1-e 1-e 0+e],[0 0 1 1-e 0+e 0+e],c2);patch([0 0 1 1-e 0+e 0+e],[0 1 1 1-e 1-e 0+e],c3);plot([0 1 1 0 0],[0 0 1 1 0]);disp('weights');
  "IW{2,1}(6,:)'" : Constant  Value=[-0.12136458297387754667884252057774574495851993560791015625;0.245074128855515771530093616092926822602748870849609375;1.0032383621174336685299977034446783363819122314453125;1.48673288863982921981232721009291708469390869140625;1.524092205330215055170128835015930235385894775390625;-3.14599198956456316267349393456242978572845458984375;-0.92344304579709668434617242382955737411975860595703125;-0.71659696819150509039531016242108307778835296630859375;2.564598622831045116043924281257204711437225341796875;-1.2510876610114409768215182339190505445003509521484375;-2.5296464836150480692822384298779070377349853515625;-0.8899425716008042552829238047706894576549530029296875;-0.53288730632954017796265588913229294121265411376953125;-1.7515635347898366180885432186187244951725006103515625;0.96152876239420859150186515762470662593841552734375;1.1514999073603122692333045051782391965389251708984375;0.7173097469275033777336147977621294558048248291015625;1.3884280426001696095994475399493239820003509521484375;-0.18901588321779250190246557394857518374919891357421875;0.01509085477404600687811875303623310173861682415008544921875]
      mask Display: e = 0.06;c1 = [120 150 230]/255;c2 = ([120 150 230]+0)/383;c3 = ([120 150 230]+128)/383;patch([0 1 1 0],[0 0 1 1],c1);patch([0 1 1 1-e 1-e 0+e],[0 0 1 1-e 0+e 0+e],c2);patch([0 0 1 1-e 0+e 0+e],[0 1 1 1-e 1-e 0+e],c3);plot([0 1 1 0 0],[0 0 1 1 0]);disp('weights');
  "IW{2,1}(7,:)'" : Constant  Value=[-0.99825808043570540828426373991533182561397552490234375;0.395191432342341053551848517599864862859249114990234375;-0.2350094964999950020168029141132137738168239593505859375;1.109293278756331435630499981925822794437408447265625;-0.91644534418474332682080785161815583705902099609375;-2.1909531762540925825533122406341135501861572265625;-2.9557855745935999181028819293715059757232666015625;-0.85874966934820162745012339655659161508083343505859375;-0.56130574084015127933611211119568906724452972412109375;2.178243849148156385808761115185916423797607421875;-1.858403927504934216585752437822520732879638671875;0.7221433377987889201676807715557515621185302734375;0.778971753058231630717500593164004385471343994140625;0.63052595385936427430095818635891191661357879638671875;0.99069209490637522019795824235188774764537811279296875;-1.972772086383116629804135300219058990478515625;1.3807830462333672283392616009223274886608123779296875;3.27820375749495074302330976934172213077545166015625;0.99841813286852409969895916219684295356273651123046875;3.09762848674741686494371606386266648769378662109375]
      mask Display: e = 0.06;c1 = [120 150 230]/255;c2 = ([120 150 230]+0)/383;c3 = ([120 150 230]+128)/383;patch([0 1 1 0],[0 0 1 1],c1);patch([0 1 1 1-e 1-e 0+e],[0 0 1 1-e 0+e 0+e],c2);patch([0 0 1 1-e 0+e 0+e],[0 1 1 1-e 1-e 0+e],c3);plot([0 1 1 0 0],[0 0 1 1 0]);disp('weights');
  "IW{2,1}(8,:)'" : Constant  Value=[-0.953955382133170104452801751904189586639404296875;0.53206594644787941206232062540948390960693359375;-0.31809051370884111609171895906911231577396392822265625;1.2689429198214183802662091693491674959659576416015625;-0.88494701597353653266253559195320121943950653076171875;-2.124342596789251302880074945278465747833251953125;-2.981479000207388541099362555542029440402984619140625;-1.069884028460427405349264518008567392826080322265625;-0.74933585130902102822147980987210758030414581298828125;1.9674124711065184012426243498339317739009857177734375;-1.7044404818984608684928616639808751642704010009765625;1.0467633545516175086476096112164668738842010498046875;1.18978837716601493212920104269869625568389892578125;0.61966152176608046975303523140610195696353912353515625;1.0446676620040007410494808937073685228824615478515625;-1.862787760122703417664524749852716922760009765625;1.299059205910026548735913820564746856689453125;3.409831012976075381715190815157257020473480224609375;0.83640287263141399609622794741881079971790313720703125;3.32949453099575709558166636270470917224884033203125]
      mask Display: e = 0.06;c1 = [120 150 230]/255;c2 = ([120 150 230]+0)/383;c3 = ([120 150 230]+128)/383;patch([0 1 1 0],[0 0 1 1],c1);patch([0 1 1 1-e 1-e 0+e],[0 0 1 1-e 0+e 0+e],c2);patch([0 0 1 1-e 0+e 0+e],[0 1 1 1-e 1-e 0+e],c3);plot([0 1 1 0 0],[0 0 1 1 0]);disp('weights');
  "IW{2,1}(9,:)'" : Constant  Value=[4.6930620898844086497092575882561504840850830078125;3.156749888514282620377571220160461962223052978515625;-1.840702818464219792105041051399894058704376220703125;-0.357046231152994553159629731453605927526950836181640625;-1.528940009510793895941560549545101821422576904296875;1.638689246590872894415724658756516873836517333984375;2.485538342938622857758446116349659860134124755859375;-1.9730202833723406996568883187137544155120849609375;-1.508609795215130500167788341059349477291107177734375;-5.31485759128989432298340034321881830692291259765625;10.8231038543341213653548038564622402191162109375;5.23169519000347182924315347918309271335601806640625;7.9575108648271157818498977576382458209991455078125;-1.7184711578232627626761086503393016755580902099609375;-6.42108777723793533453999771154485642910003662109375;3.266886668560809336980810257955454289913177490234375;-14.6132398600836435065275509259663522243499755859375;-3.726687276355495015423002769239246845245361328125;-6.4179178254200710540544605464674532413482666015625;-4.56225472315612545770591168547980487346649169921875]
      mask Display: e = 0.06;c1 = [120 150 230]/255;c2 = ([120 150 230]+0)/383;c3 = ([120 150 230]+128)/383;patch([0 1 1 0],[0 0 1 1],c1);patch([0 1 1 1-e 1-e 0+e],[0 0 1 1-e 0+e 0+e],c2);patch([0 0 1 1-e 0+e 0+e],[0 1 1 1-e 1-e 0+e],c3);plot([0 1 1 0 0],[0 0 1 1 0]);disp('weights');
  Mux : Mux  Inputs=10
      mask Display: e = 0.06;c1 = [120 150 230]/255;c2 = ([120 150 230]+0)/383;c3 = ([120 150 230]+128)/383;patch([0 1 1 0],[0 0 1 1],c1);patch([0 1 1 1-e 1-e 0+e],[0 0 1 1-e 0+e 0+e],c2);patch([0 0 1 1-e 0+e 0+e],[0 1 1 1-e 1-e 0+e],c3);plot([0 1 1 0 0],[0 0 1 1 0]);disp('Mux');
  dotprod{1..10} (10 alike) : neural/Weight Functions/dotprod
  "lz{2,1}" : Outport
      mask Display: e = 0.06;c1 = [120 230 180]/255;c2 = ([120 230 180]+0)/(256+128);c3 = ([120 230 180]+128)/(256+128);patch([0 1 1 0],[0 0 1 1],c1);patch([0 1 1 1-e 1-e 0+e],[0 0 1 1-e 0+e 0+e],c2);patch([0 0 1 1-e 0+e 0+e],[0 1 1 1-e 1-e 0+e],c3);plot([0 1 1 0 0],[0 0 1 1 0]);
  wires:
  "IW{2,1}(1,:)'"/1 -> dotprod1/1
  "ad{2,1}"/1 -> dotprod1/2, dotprod2/2, dotprod3/2, dotprod4/2, dotprod5/2, dotprod6/2, dotprod7/2, dotprod8/2, dotprod9/2, dotprod10/2
  dotprod1/1 -> Mux/1
  "IW{2,1}(2,:)'"/1 -> dotprod2/1
  dotprod2/1 -> Mux/2
  "IW{2,1}(3,:)'"/1 -> dotprod3/1
  dotprod3/1 -> Mux/3
  "IW{2,1}(4,:)'"/1 -> dotprod4/1
  dotprod4/1 -> Mux/4
  "IW{2,1}(5,:)'"/1 -> dotprod5/1
  dotprod5/1 -> Mux/5
  "IW{2,1}(6,:)'"/1 -> dotprod6/1
  dotprod6/1 -> Mux/6
  "IW{2,1}(7,:)'"/1 -> dotprod7/1
  dotprod7/1 -> Mux/7
  "IW{2,1}(8,:)'"/1 -> dotprod8/1
  dotprod8/1 -> Mux/8
  "IW{2,1}(9,:)'"/1 -> dotprod9/1
  dotprod9/1 -> Mux/9
  "IW{2,1}(10,:)'"/1 -> dotprod10/1
  dotprod10/1 -> Mux/10
  Mux/1 -> "lz{2,1}"/1

== system mi_modelo_MI/FFNN FluxRotor/Layer 3/Delays 1 ==
  "p{3}" : Inport  PortDimensions=10
      mask Display: e = 0.06;c1 = [120 230 180]/255;c2 = ([120 230 180]+0)/(256+128);c3 = ([120 230 180]+128)/(256+128);patch([0 1 1 0],[0 0 1 1],c1);patch([0 1 1 1-e 1-e 0+e],[0 0 1 1-e 0+e 0+e],c2);patch([0 0 1 1-e 0+e 0+e],[0 1 1 1-e 1-e 0+e],c3);plot([0 1 1 0 0],[0 0 1 1 0]);
  mux : Mux  Inputs=1
      mask Display: e = 0.06;c1 = [120 150 230]/255;c2 = ([120 150 230]+0)/383;c3 = ([120 150 230]+128)/383;patch([0 1 1 0],[0 0 1 1],c1);patch([0 1 1 1-e 1-e 0+e],[0 0 1 1-e 0+e 0+e],c2);patch([0 0 1 1-e 0+e 0+e],[0 1 1 1-e 1-e 0+e],c3);plot([0 1 1 0 0],[0 0 1 1 0]);disp('Mux')
  "pd{3,2}" : Outport
      mask Display: e = 0.06;c1 = [120 230 180]/255;c2 = ([120 230 180]+0)/(256+128);c3 = ([120 230 180]+128)/(256+128);patch([0 1 1 0],[0 0 1 1],c1);patch([0 1 1 1-e 1-e 0+e],[0 0 1 1-e 0+e 0+e],c2);patch([0 0 1 1-e 0+e 0+e],[0 1 1 1-e 1-e 0+e],c3);plot([0 1 1 0 0],[0 0 1 1 0]);
  wires:
  "p{3}"/1 -> mux/1
  mux/1 -> "pd{3,2}"/1

== system mi_modelo_MI/FFNN FluxRotor/Layer 3/LW{3,2} ==
  "ad{3,2}" : Inport  PortDimensions=10
      mask Display: e = 0.06;c1 = [120 230 180]/255;c2 = ([120 230 180]+0)/(256+128);c3 = ([120 230 180]+128)/(256+128);patch([0 1 1 0],[0 0 1 1],c1);patch([0 1 1 1-e 1-e 0+e],[0 0 1 1-e 0+e 0+e],c2);patch([0 0 1 1-e 0+e 0+e],[0 1 1 1-e 1-e 0+e],c3);plot([0 1 1 0 0],[0 0 1 1 0]);
  "IW{3,2}(1,:)'" : Constant  Value=[1.121065594753122507398757079499773681163787841796875;0.223039929807466841271690327630494721233844757080078125;0.80262920022987238599654347126488573849201202392578125;0.677855082879858183986243602703325450420379638671875;-0.38329938201300939315530058593139983713626861572265625;-0.1877222056562998508955075749327079392969608306884765625;-4.78861277668787632677549481741152703762054443359375;4.23781657772022679608880935120396316051483154296875;-0.27232736349400032960232920231646858155727386474609375;0.403037582151535456187474437683704309165477752685546875]
      mask Display: e = 0.06;c1 = [120 150 230]/255;c2 = ([120 150 230]+0)/383;c3 = ([120 150 230]+128)/383;patch([0 1 1 0],[0 0 1 1],c1);patch([0 1 1 1-e 1-e 0+e],[0 0 1 1-e 0+e 0+e],c2);patch([0 0 1 1-e 0+e 0+e],[0 1 1 1-e 1-e 0+e],c3);plot([0 1 1 0 0],[0 0 1 1 0]);disp('weights');
  "IW{3,2}(2,:)'" : Constant  Value=[0.258119357726853682066803230554796755313873291015625;-1.120210088000675341390888206660747528076171875;0.9682162345519482737898897539707832038402557373046875;0.8736555013585010076582193505601026117801666259765625;-0.2441636052810340073992989573525846935808658599853515625;-0.7351559721308633665870502227335236966609954833984375;2.29438633243280865059432471753098070621490478515625;-2.61474775001114334571639119531027972698211669921875;0.1336349675366431399847755301379947923123836517333984375;-0.08587047177098046379928319993268814869225025177001953125]
      mask Display: e = 0.06;c1 = [120 150 230]/255;c2 = ([120 150 230]+0)/383;c3 = ([120 150 230]+128)/383;patch([0 1 1 0],[0 0 1 1],c1);patch([0 1 1 1-e 1-e 0+e],[0 0 1 1-e 0+e 0+e],c2);patch([0 0 1 1-e 0+e 0+e],[0 1 1 1-e 1-e 0+e],c3);plot([0 1 1 0 0],[0 0 1 1 0]);disp('weights');
  Mux : Mux  Inputs=2
      mask Display: e = 0.06;c1 = [120 150 230]/255;c2 = ([120 150 230]+0)/383;c3 = ([120 150 230]+128)/383;patch([0 1 1 0],[0 0 1 1],c1);patch([0 1 1 1-e 1-e 0+e],[0 0 1 1-e 0+e 0+e],c2);patch([0 0 1 1-e 0+e 0+e],[0 1 1 1-e 1-e 0+e],c3);plot([0 1 1 0 0],[0 0 1 1 0]);disp('Mux');
  dotprod1 : neural/Weight Functions/dotprod
  dotprod2 : neural/Weight Functions/dotprod
  "lz{3,2}" : Outport
      mask Display: e = 0.06;c1 = [120 230 180]/255;c2 = ([120 230 180]+0)/(256+128);c3 = ([120 230 180]+128)/(256+128);patch([0 1 1 0],[0 0 1 1],c1);patch([0 1 1 1-e 1-e 0+e],[0 0 1 1-e 0+e 0+e],c2);patch([0 0 1 1-e 0+e 0+e],[0 1 1 1-e 1-e 0+e],c3);plot([0 1 1 0 0],[0 0 1 1 0]);
  wires:
  "IW{3,2}(1,:)'"/1 -> dotprod1/1
  "ad{3,2}"/1 -> dotprod1/2, dotprod2/2
  dotprod1/1 -> Mux/1
  "IW{3,2}(2,:)'"/1 -> dotprod2/1
  dotprod2/1 -> Mux/2
  Mux/1 -> "lz{3,2}"/1

== system mi_modelo_MI/FFNN WR/Layer 1/Delays 1 ==
  "p{1}" : Inport  PortDimensions=4
      mask Display: e = 0.06;c1 = [120 230 180]/255;c2 = ([120 230 180]+0)/(256+128);c3 = ([120 230 180]+128)/(256+128);patch([0 1 1 0],[0 0 1 1],c1);patch([0 1 1 1-e 1-e 0+e],[0 0 1 1-e 0+e 0+e],c2);patch([0 0 1 1-e 0+e 0+e],[0 1 1 1-e 1-e 0+e],c3);plot([0 1 1 0 0],[0 0 1 1 0]);
  mux : Mux  Inputs=1
      mask Display: e = 0.06;c1 = [120 150 230]/255;c2 = ([120 150 230]+0)/383;c3 = ([120 150 230]+128)/383;patch([0 1 1 0],[0 0 1 1],c1);patch([0 1 1 1-e 1-e 0+e],[0 0 1 1-e 0+e 0+e],c2);patch([0 0 1 1-e 0+e 0+e],[0 1 1 1-e 1-e 0+e],c3);plot([0 1 1 0 0],[0 0 1 1 0]);disp('Mux')
  "pd{1,1}" : Outport
      mask Display: e = 0.06;c1 = [120 230 180]/255;c2 = ([120 230 180]+0)/(256+128);c3 = ([120 230 180]+128)/(256+128);patch([0 1 1 0],[0 0 1 1],c1);patch([0 1 1 1-e 1-e 0+e],[0 0 1 1-e 0+e 0+e],c2);patch([0 0 1 1-e 0+e 0+e],[0 1 1 1-e 1-e 0+e],c3);plot([0 1 1 0 0],[0 0 1 1 0]);
  wires:
  "p{1}"/1 -> mux/1
  mux/1 -> "pd{1,1}"/1
